simulink model "colas_lin"  (Simulink 2.09)
settings: Solver=ode45  StartTime=0.0  StopTime=100  MaxStep=10  RelTol=1e-5  AbsTol=1e-5
values from neighbouring files (symbols this model uses):
  A = [ -5.131e-3 0 0 0 0; 0 -7.366e-2 0 0 0; 0 0 -1.829e-1 0 0 ... (first row only)    [cola_commands.m]
  B = 0.5    [cola4.m]    (also in cola4_F1.m; cola_commands.m = [-.629 .624; .055 -0.172; 0.030 -0.108; cola_db.m; cola_dv.m = Bs+(MB-MBs)*KcB)
  C = [-0.7223 -0.5170 0.3386 -0.1633e-1 0.1121 ... (first row only)    [cola_commands.m]
  D = 0.5    [cola4.m]    (also in cola4_F1.m; cola_commands.m = [ 0 0; 0 0]; cola_db.m; cola_dv.m)
settings Model: SaveTime=off  SaveOutput=off  ConsistencyChecking=off  RTWTemplateMakefile=grt_unix.tmf

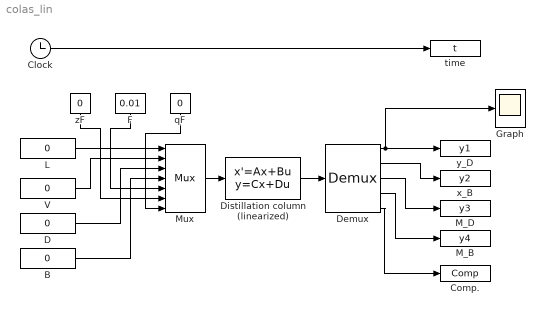
== system colas_lin ==
  B : Constant  Value=0
  Clock : Clock
  Comp. : ToWorkspace  VariableName=Comp  SampleTime=0
      settings: Buffer=1000
  D : Constant  Value=0
  Demux : Demux  Outputs=[1,1,1,1,41]
  Distillation column (linearized) : StateSpace  A=A  B=B  C=C  D=D  X0=0
  F : Constant  Orientation=down  Value=0.01
  Graph : Scope
      settings: TickLabels=on  TimeRange=100  YMin=-0.01  YMax=0.2  SaveToWorkspace=off  SaveName=ScopeData
  L : Constant  Value=0
  M_B : ToWorkspace  VariableName=y4  SampleTime=0
      settings: Buffer=1000
  M_D : ToWorkspace  VariableName=y3  SampleTime=0
      settings: Buffer=1000
  Mux : Mux  Inputs=7
  V : Constant  Value=0
  qF : Constant  Orientation=down  Value=0
  time : ToWorkspace  VariableName=t  SampleTime=0
      settings: Buffer=1000
  x_B : ToWorkspace  VariableName=y2  SampleTime=0
      settings: Buffer=1000
  y_D : ToWorkspace  VariableName=y1  SampleTime=0
      settings: Buffer=1000
  zF : Constant  Orientation=down  Value=0
  wires:
  qF/1 -> Mux/7
  Demux/1 -> Graph/1, y_D/1
  Mux/1 -> Distillation column (linearized)/1
  Demux/2 -> x_B/1
  Distillation column (linearized)/1 -> Demux/1
  Clock/1 -> time/1
  zF/1 -> Mux/6
  V/1 -> Mux/2
  F/1 -> Mux/5
  Demux/5 -> Comp./1
  Demux/4 -> M_B/1
  Demux/3 -> M_D/1
  B/1 -> Mux/4
  D/1 -> Mux/3
  L/1 -> Mux/1
